simulink model "Actuators_UltraStick25e"  (R2016b)
settings: Solver=VariableStepAuto  StartTime=0.0  StopTime=10.0  RelTol=1e-3
undefined symbols (not defined in the file): AC
libraries: Actuator_Lib x6
settings Model: Creator=UAVLAB  LastModifiedBy=UAVLAB

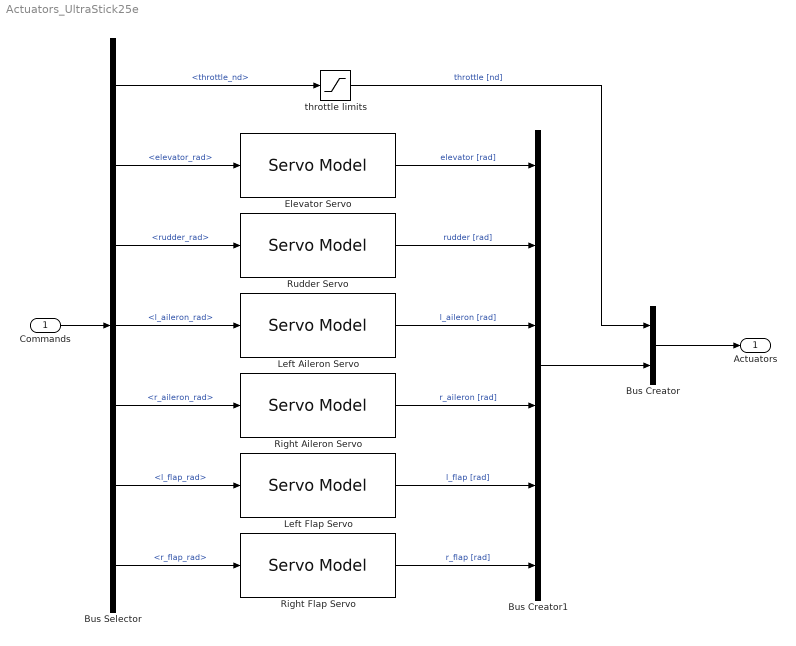
== system Actuators_UltraStick25e ==
  Commands : Inport  OutDataTypeStr=Bus: Commands
  Bus Creator : BusCreator  Inputs=2  OutDataTypeStr=Bus: Actuators
      settings: InheritFromInputs=off
  Bus Creator1 : BusCreator  Inputs=6  OutDataTypeStr=Bus: CtrlSurf
      settings: InheritFromInputs=off
  Bus Selector : BusSelector  OutputSignals=throttle_nd,elevator_rad,rudder_rad,l_aileron_rad,r_aileron_rad,l_flap_rad,r_flap_rad
  Elevator Servo : Actuator_Lib/Servo Model  freq=AC.Actuator.elevator.BW  RL=AC.Actuator.elevator.RateLim  POS_hi=AC.Actuator.elevator.PosLim  POS_lo=AC.Actuator.elevator.NegLim
  Left Aileron Servo : Actuator_Lib/Servo Model  freq=AC.Actuator.l_aileron.BW  RL=AC.Actuator.l_aileron.RateLim  POS_hi=AC.Actuator.l_aileron.PosLim  POS_lo=AC.Actuator.l_aileron.NegLim
  Left Flap Servo : Actuator_Lib/Servo Model  freq=AC.Actuator.l_flap.BW  RL=AC.Actuator.l_flap.RateLim  POS_hi=AC.Actuator.l_flap.PosLim  POS_lo=AC.Actuator.l_flap.NegLim
  Right Aileron Servo : Actuator_Lib/Servo Model  freq=AC.Actuator.r_aileron.BW  RL=AC.Actuator.r_aileron.RateLim  POS_hi=AC.Actuator.r_aileron.PosLim  POS_lo=AC.Actuator.r_aileron.NegLim
  Right Flap Servo : Actuator_Lib/Servo Model  freq=AC.Actuator.l_flap.BW  RL=AC.Actuator.l_flap.RateLim  POS_hi=AC.Actuator.l_flap.PosLim  POS_lo=AC.Actuator.l_flap.NegLim
  Rudder Servo : Actuator_Lib/Servo Model  freq=AC.Actuator.rudder.BW  RL=AC.Actuator.rudder.RateLim  POS_hi=AC.Actuator.rudder.PosLim  POS_lo=AC.Actuator.rudder.NegLim
  throttle limits : Saturate  UpperLimit=AC.Actuator.throttle.PosLim  LowerLimit=AC.Actuator.throttle.NegLim
  Actuators : Outport  OutDataTypeStr=Bus: Actuators
  wires:
  Bus Creator1/1 -> Bus Creator/2
  Bus Creator/1 -> Actuators/1
  Commands/1 -> Bus Selector/1
  Bus Selector/1 -> throttle limits/1  "<throttle_nd>"
  Bus Selector/2 -> Elevator Servo/1  "<elevator_rad>"
  Elevator Servo/1 -> Bus Creator1/1  "elevator [rad]"
  Bus Selector/3 -> Rudder Servo/1  "<rudder_rad>"
  Bus Selector/4 -> Left Aileron Servo/1  "<l_aileron_rad>"
  Left Aileron Servo/1 -> Bus Creator1/3  "l_aileron [rad]"
  Bus Selector/6 -> Left Flap Servo/1  "<l_flap_rad>"
  Left Flap Servo/1 -> Bus Creator1/5  "l_flap [rad]"
  Right Aileron Servo/1 -> Bus Creator1/4  "r_aileron [rad]"
  Right Flap Servo/1 -> Bus Creator1/6  "r_flap [rad]"
  Bus Selector/7 -> Right Flap Servo/1  "<r_flap_rad>"
  throttle limits/1 -> Bus Creator/1  "throttle [nd]"
  Rudder Servo/1 -> Bus Creator1/2  "rudder [rad]"
  Bus Selector/5 -> Right Aileron Servo/1  "<r_aileron_rad>"
